simulink model "Bicyle_Simulink_Model"  (R2024a)
settings: Solver=ode4  StartTime=0.0  StopTime=10.0  FixedStep=0.1  RelTol=1e-3
undefined symbols (not defined in the file): Acl, Acl_steer, Ass, Bcl, Bcl_steer, Bss, c, Ccl, Ccl_steer, Css, Dcl, Dcl_steer, Dss, K, K_steer, lambda, v, w
settings Model: Creator=Vipuls  LastModifiedBy=Vipuls

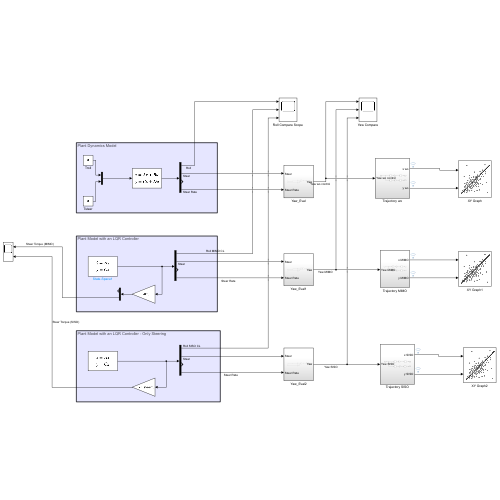
[thumbnail: Simulink's stored preview of the top-level diagram]
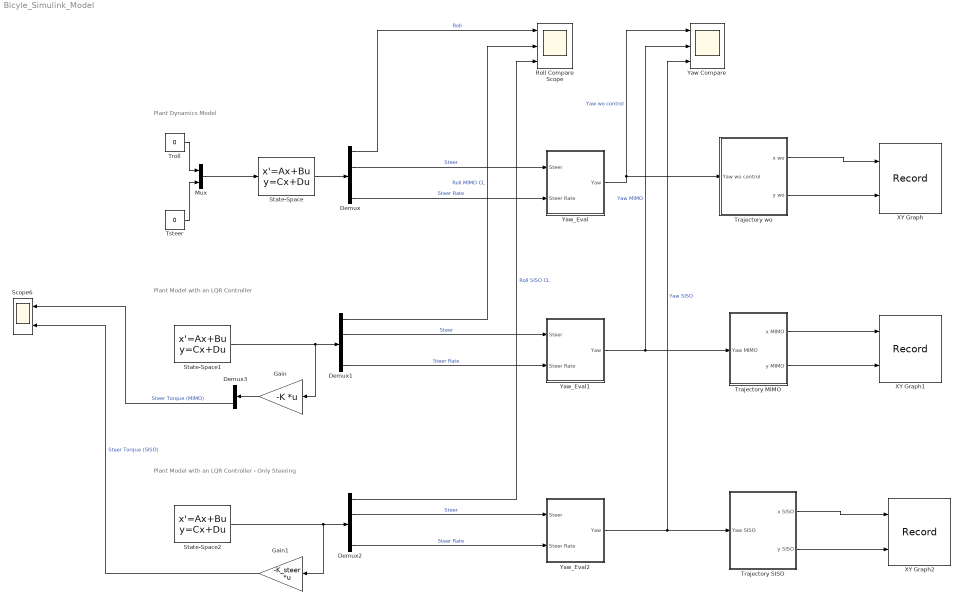
== system Bicyle_Simulink_Model ==
  note: Plant Dynamics Model
  note: Plant Model with an LQR Controller
  note: Plant Model with an LQR Controller - Only Steering
  Demux : Demux
  Demux1 : Demux
  Demux2 : Demux
  Demux3 : Demux  Outputs=2
  Gain : Gain  Gain=-K  Multiplication=Matrix(K*u)
  Gain1 : Gain  Gain=-K_steer  Multiplication=Matrix(K*u)
  Mux : Mux  Inputs=2
  Roll Compare Scope : Scope  NumInputPorts=3
  Scope6 : Scope  NumInputPorts=2
  State-Space : StateSpace  A=Ass  B=Bss  C=Css  D=Dss  InitialCondition=[0.15,0,1.5,0]
  State-Space1 : StateSpace  A=Acl  B=Bcl  C=Ccl  D=Dcl  InitialCondition=[0.15,0,1.5,0]
  State-Space2 : StateSpace  A=Acl_steer  B=Bcl_steer  C=Ccl_steer  D=Dcl_steer  InitialCondition=[0.15,0,1.5,0]
  Trajectory MIMO : Subsystem
  Trajectory SISO : Subsystem
  Trajectory wo : Subsystem
  Troll : Constant  Value=0
  Tsteer : Constant  Value=0
  XY Graph : Record  FileSettingsInternal="{\"entries\":[{\"content\":{\"excelSettings\":{\"content\":{},\"type\":\"Streamout.ExcelSettings\"}},\"type\":\"Streamout.FileSettingStorage\",\"uuid\":\"\"}],\"packageUris\":[\"http:\\/\\/schema.mathworks.com\\/mf0\\/streamout_blocks\\/R2020a\"],\"version\":\"1.0\"}"  Layout=[1 1]  SignalsInternal="{\"entries\":[{\"content\":{\"signals\":[{\"content\":{\"blockPath\":[],\"dimensions\":[1],\"domain\":\"\",\"lineColor\":\"#b746ff\",\"port\":1,\"sid\":[\"\"],\"signalID\":1,\"signalName\":\"Trajectory wo:1\"},\"type\":\"RecordBlkView.Signal\",\"uuid\":\"\"},{\"content\":{\"blockPath\":[],\"dimensions\":[1],\"domain\":\"\",\"lineColor\":\"#b746ff\",\"port\":2,\"sid\":[\"\"],\"signalID\":2,\"signalName\":\"Trajectory wo:2\"},\"type\":\"RecordBlkView.Signal\",\"uuid\":\"\"}]},\"type\":\"RecordBlkView.InputSignals\",\"uuid\":\"\"}],\"packageUris\":[\"http:\\/\\/schema.mathworks.com\\/mf0\\/streamout_blocks\\/R2020a\"],\"version\":\"1.0\"}"  VisualizationBindings="{\"xyplotplugin\":{\"info\":[{\"series\":[{\"bindingParametersList\":[{\"parameter\":\"X-Axis\",\"signalID\":223,\"signalName\":\"XandY:1\"},{\"parameter\":\"Y-Axis\",\"signalID\":227,\"signalName\":\"XandY:2\"}],\"seriesID\":0}],\"subplotID\":1}]}}"  CompatibilityTag=XY
  XY Graph1 : Record  FileSettingsInternal="{\"entries\":[{\"content\":{\"excelSettings\":{\"content\":{},\"type\":\"Streamout.ExcelSettings\"}},\"type\":\"Streamout.FileSettingStorage\",\"uuid\":\"\"}],\"packageUris\":[\"http:\\/\\/schema.mathworks.com\\/mf0\\/streamout_blocks\\/R2020a\"],\"version\":\"1.0\"}"  Layout=[1 1]  SignalsInternal="{\"entries\":[{\"content\":{\"signals\":[{\"content\":{\"blockPath\":[],\"dimensions\":[1],\"domain\":\"\",\"lineColor\":\"#64d413\",\"plots\":[ 1 ],\"port\":1,\"sid\":[\"\"],\"signalID\":1,\"signalName\":\"Trajectory MIMO:1\"},\"type\":\"RecordBlkView.Signal\",\"uuid\":\"\"},{\"content\":{\"blockPath\":[],\"dimensions\":[1],\"domain\":\"\",\"lineColor\":\"#64d413\",\"plots\":[ 1 ],\"port\":2,\"sid\":[\"\"],\"signalID\":2,\"signalName\":\"Trajectory MIMO:2\"},\"type\":\"RecordBlkView.Signal\",\"uuid\":\"\"}]},\"type\":\"RecordBlkView.InputSignals\",\"uuid\":\"\"}],\"packageUris\":[\"http:\\/\\/schema.mathworks.com\\/mf0\\/streamout_blocks\\/R2020a\"],\"version\":\"1.0\"}"  VisualizationBindings="{\"xyplotplugin\":{\"info\":[{\"series\":[{\"bindingParametersList\":[{\"parameter\":\"X-Axis\",\"signalID\":1,\"signalName\":\"Trajectory MIMO:1\"},{\"parameter\":\"Y-Axis\",\"signalID\":2,\"signalName\":\"Trajectory MIMO:2\"}],\"seriesID\":0}],\"subplotID\":1}]}}"  CompatibilityTag=XY
  XY Graph2 : Record  FileSettingsInternal="{\"entries\":[{\"content\":{\"excelSettings\":{\"content\":{},\"type\":\"Streamout.ExcelSettings\"}},\"type\":\"Streamout.FileSettingStorage\",\"uuid\":\"\"}],\"packageUris\":[\"http:\\/\\/schema.mathworks.com\\/mf0\\/streamout_blocks\\/R2020a\"],\"version\":\"1.0\"}"  Layout=[1 1]  SignalsInternal="{\"entries\":[{\"content\":{\"signals\":[{\"content\":{\"blockPath\":[],\"dimensions\":[1],\"domain\":\"\",\"lineColor\":\"#ff13a6\",\"plots\":[ 1 ],\"port\":1,\"sid\":[\"\"],\"signalID\":1,\"signalName\":\"Trajectory SISO:1\"},\"type\":\"RecordBlkView.Signal\",\"uuid\":\"\"},{\"content\":{\"blockPath\":[],\"dimensions\":[1],\"domain\":\"\",\"lineColor\":\"#ff13a6\",\"plots\":[ 1 ],\"port\":2,\"sid\":[\"\"],\"signalID\":2,\"signalName\":\"Trajectory SISO:2\"},\"type\":\"RecordBlkView.Signal\",\"uuid\":\"\"}]},\"type\":\"RecordBlkView.InputSignals\",\"uuid\":\"\"}],\"packageUris\":[\"http:\\/\\/schema.mathworks.com\\/mf0\\/streamout_blocks\\/R2020a\"],\"version\":\"1.0\"}"  VisualizationBindings="{\"xyplotplugin\":{\"info\":[{\"series\":[{\"bindingParametersList\":[{\"parameter\":\"X-Axis\",\"signalID\":1,\"signalName\":\"Trajectory SISO:1\"},{\"parameter\":\"Y-Axis\",\"signalID\":2,\"signalName\":\"Trajectory SISO:2\"}],\"seriesID\":0}],\"subplotID\":1}]}}"  CompatibilityTag=XY
  Yaw Compare : Scope  NumInputPorts=3
  Yaw_Eval : Subsystem
  Yaw_Eval1 : Subsystem
  Yaw_Eval2 : Subsystem
  wires:
  Mux/1 -> State-Space/1
  State-Space/1 -> Demux/1
  Demux/1 -> Roll Compare Scope/1  "Roll"
  Troll/1 -> Mux/1
  Tsteer/1 -> Mux/2
  Demux1/1 -> Roll Compare Scope/2  "Roll MIMO CL"
  Demux1/4 -> Yaw_Eval1/2(Steer Rate)  "Steer Rate"
  State-Space1/1 -> Gain/1, Demux1/1
  Demux2/1 -> Roll Compare Scope/3  "Roll SISO CL"
  Demux2/2 -> Yaw_Eval2/1(Steer)  "Steer"
  Demux2/4 -> Yaw_Eval2/2(Steer Rate)  "Steer Rate"
  State-Space2/1 -> Demux2/1, Gain1/1
  Gain/1 -> Demux3/1
  Demux3/2 -> Scope6/1  "Steer Torque (MIMO)"
  Gain1/1 -> Scope6/2  "Steer Torque (SISO)"
  Demux/2 -> Yaw_Eval/1(Steer)  "Steer"
  Demux/4 -> Yaw_Eval/2(Steer Rate)  "Steer Rate"
  Demux1/2 -> Yaw_Eval1/1(Steer)  "Steer"
  Yaw_Eval/1(Yaw) -> Yaw Compare/1, Trajectory wo/1(Yaw wo control)  "Yaw wo control"
  Yaw_Eval1/1(Yaw) -> Yaw Compare/2, Trajectory MIMO/1(Yaw MIMO)  "Yaw MIMO"
  Yaw_Eval2/1(Yaw) -> Yaw Compare/3, Trajectory SISO/1(Yaw SISO)  "Yaw SISO"
  Trajectory wo/1(x wo) -> XY Graph/1
  Trajectory wo/2(y wo) -> XY Graph/2
  Trajectory MIMO/1(x MIMO) -> XY Graph1/1
  Trajectory MIMO/2(y MIMO) -> XY Graph1/2
  Trajectory SISO/1(x SISO) -> XY Graph2/1
  Trajectory SISO/2(y SISO) -> XY Graph2/2

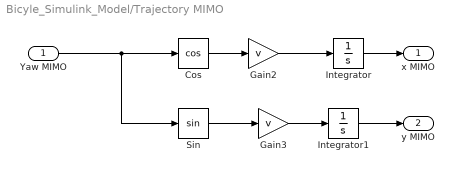
== system Bicyle_Simulink_Model/Trajectory MIMO ==
  Yaw MIMO : Inport
  Cos : Trigonometry  Operator=cos
  Gain2 : Gain  Gain=v
  Gain3 : Gain  Gain=v
  Integrator : Integrator
  Integrator1 : Integrator
  Sin : Trigonometry
  x MIMO : Outport
  y MIMO : Outport  Port=2
  wires:
  Sin/1 -> Gain3/1
  Cos/1 -> Gain2/1
  Gain3/1 -> Integrator1/1
  Gain2/1 -> Integrator/1
  Yaw MIMO/1 -> Sin/1, Cos/1
  Integrator/1 -> x MIMO/1
  Integrator1/1 -> y MIMO/1

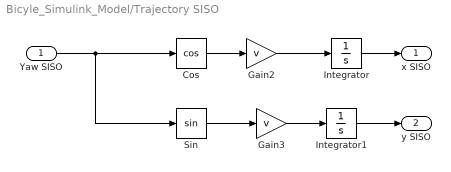
== system Bicyle_Simulink_Model/Trajectory SISO ==
  Yaw SISO : Inport
  Cos : Trigonometry  Operator=cos
  Gain2 : Gain  Gain=v
  Gain3 : Gain  Gain=v
  Integrator : Integrator
  Integrator1 : Integrator
  Sin : Trigonometry
  x SISO : Outport
  y SISO : Outport  Port=2
  wires:
  Sin/1 -> Gain3/1
  Cos/1 -> Gain2/1
  Gain3/1 -> Integrator1/1
  Gain2/1 -> Integrator/1
  Yaw SISO/1 -> Sin/1, Cos/1
  Integrator/1 -> x SISO/1
  Integrator1/1 -> y SISO/1

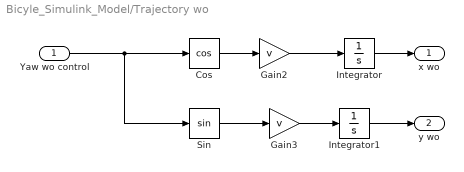
== system Bicyle_Simulink_Model/Trajectory wo ==
  Yaw wo control : Inport
  Cos : Trigonometry  Operator=cos
  Gain2 : Gain  Gain=v
  Gain3 : Gain  Gain=v
  Integrator : Integrator
  Integrator1 : Integrator
  Sin : Trigonometry
  x wo : Outport
  y wo : Outport  Port=2
  wires:
  Sin/1 -> Gain3/1
  Cos/1 -> Gain2/1
  Gain3/1 -> Integrator1/1
  Gain2/1 -> Integrator/1
  Yaw wo control/1 -> Sin/1, Cos/1
  Integrator/1 -> x wo/1
  Integrator1/1 -> y wo/1

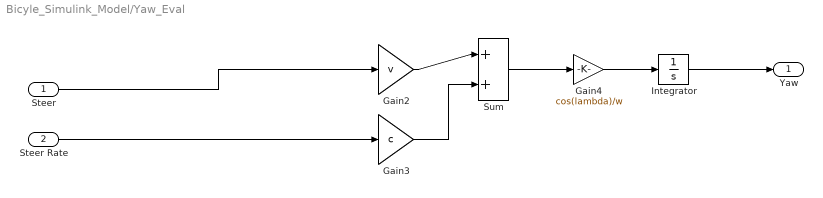
== system Bicyle_Simulink_Model/Yaw_Eval ==
  Steer : Inport
  Steer Rate : Inport  Port=2
  Gain2 : Gain  Gain=v
  Gain3 : Gain  Gain=c
  Gain4 : Gain  Gain=cos(lambda)/w
  Integrator : Integrator
  Sum : Sum  Inputs=|++
  Yaw : Outport
  wires:
  Sum/1 -> Gain4/1
  Gain4/1 -> Integrator/1
  Integrator/1 -> Yaw/1
  Gain3/1 -> Sum/2
  Steer Rate/1 -> Gain3/1
  Gain2/1 -> Sum/1
  Steer/1 -> Gain2/1

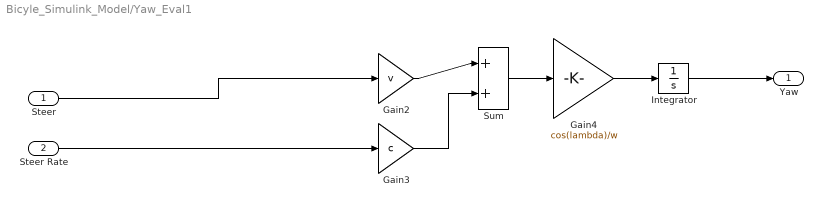
== system Bicyle_Simulink_Model/Yaw_Eval1 ==
  Steer : Inport
  Steer Rate : Inport  Port=2
  Gain2 : Gain  Gain=v
  Gain3 : Gain  Gain=c
  Gain4 : Gain  Gain=cos(lambda)/w
  Integrator : Integrator
  Sum : Sum  Inputs=|++
  Yaw : Outport
  wires:
  Sum/1 -> Gain4/1
  Gain4/1 -> Integrator/1
  Integrator/1 -> Yaw/1
  Gain3/1 -> Sum/2
  Steer Rate/1 -> Gain3/1
  Gain2/1 -> Sum/1
  Steer/1 -> Gain2/1

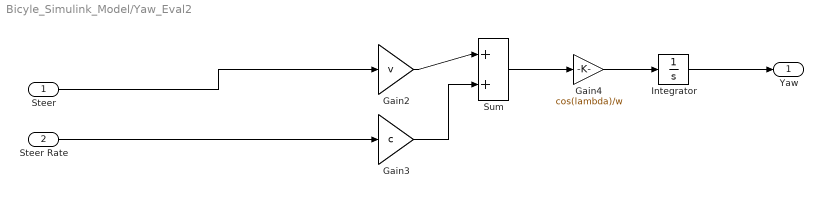
== system Bicyle_Simulink_Model/Yaw_Eval2 ==
  Steer : Inport
  Steer Rate : Inport  Port=2
  Gain2 : Gain  Gain=v
  Gain3 : Gain  Gain=c
  Gain4 : Gain  Gain=cos(lambda)/w
  Integrator : Integrator
  Sum : Sum  Inputs=|++
  Yaw : Outport
  wires:
  Sum/1 -> Gain4/1
  Gain4/1 -> Integrator/1
  Integrator/1 -> Yaw/1
  Gain3/1 -> Sum/2
  Steer Rate/1 -> Gain3/1
  Gain2/1 -> Sum/1
  Steer/1 -> Gain2/1
